simulink model "CruiseControl"  (R2020a)
settings: Solver=FixedStepAuto  StartTime=0.0  StopTime=300  FixedStep=0.01  RelTol=1e-3
settings Model: Creator=Lenovo  LastModifiedBy=Lenovo

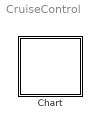
== system CruiseControl ==
  Chart : Stateflow chart  TreatAsAtomicUnit=on

== stateflow chart CruiseControl/Chart ==
  settings: updateMethod=CONTINUOUS
  state B21
    du:
    v_dot = -t - 2.5;
    x_dot = 0;
    t_dot = 1;
  state B22
    du:
    v_dot = -5;
    x_dot = 0;
    t_dot = 0;
  state B11
    du:
    v_dot = -t - 1.2;
    x_dot = 0;
    t_dot = 0.5;
  state B12
    du:
    v_dot = -2.5;
    x_dot = 0;
    t_dot = 0;
  state N
    du:
    v_dot = -0.001 * x - 0.052 * v;
    x_dot = v;
    t_dot = 0;
  state A
    du:
    v_dot = 1.5;
    x_dot = 0;
    t_dot = 0;
  B21 -> B22 [order 1] : [t >= 2.5 && 15 <= v && v <= 40]
  B12 -> B21 [order 1] : [18 <= v && v <= 20 && t >= 1.3]{t = 0}
  B22 -> B11 : [15 <= v && v <= 16 && t >= 2.5]{t = 0}
  B11 -> B21 [order 1] : [18 <= v && v <= 20 && 0 <= t && t <= 1.3]{t = 0}
  B21 -> B11 [order 2] : [15 <= v && v <= 16 && 0 <= t && t <= 2.5]{t = 0}
  B11 -> B12 [order 2] : [t >= 1.3 && 5 <= v && v <= 20]
  B12 -> N [order 2] : [5 <= v && v <= 11 && t >= 1.3]{x = 0}
  N -> B11 [order 1] : [13 <= v && v <= 15 && -500 <= x && x <= 500]{t = 0}
  B11 -> N [order 3] : [5 <= v && v <= 11 && 0 <= t && t <= 1.3]{x = 0}
  (default) -> N : {v = 10;
      |  t = 0;
      |  x = 0;}
  A -> N : [-6 <= v && v <= -5 && -500 <= x && x <= 500]{x = 0}
  N -> A [order 2] : [-15 <= v && v <= -14 && -500 <= x && x <= 500]
  data: x local; t local; v local
  data x settings: updateMethod=SF_CONTINUOUS_TIME_DATA
  data t settings: updateMethod=SF_CONTINUOUS_TIME_DATA
  data v settings: updateMethod=SF_CONTINUOUS_TIME_DATA
